simulink model "LQR_s_inv_int"  (R2023b)
settings: Solver=VariableStepAuto  StartTime=0.0  StopTime=10  RelTol=1e-14  AbsTol=1e-20
values from neighbouring files (symbols this model uses):
  K = [k1 k2 ki]    [WP2.m]
undefined symbols (not defined in the file or in its folder): Disturbo
settings Model: Creator=giova  LastModifiedBy=Principale

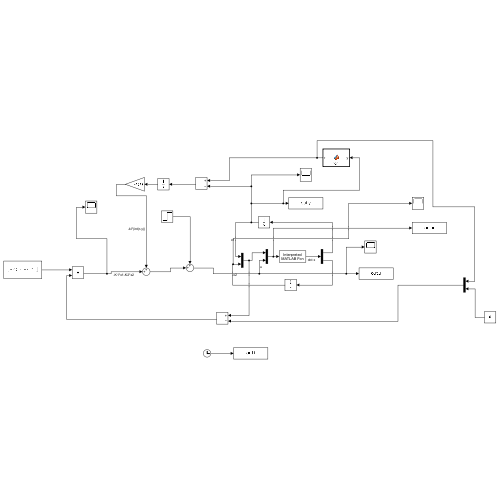
[thumbnail: Simulink's stored preview of the top-level diagram]
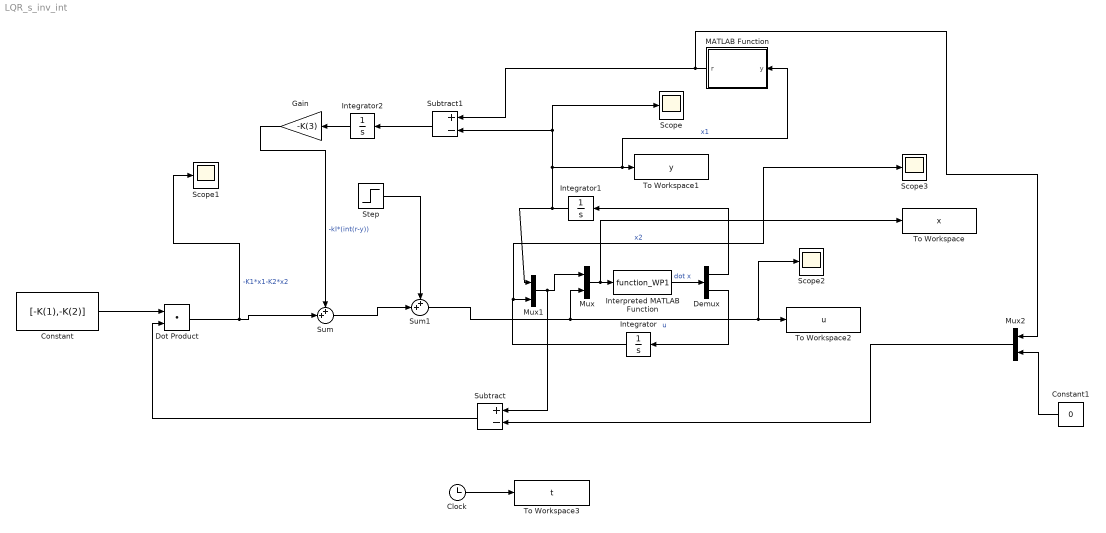
== system LQR_s_inv_int ==
  Clock : Clock
  Constant : Constant  Value=[-K(1),-K(2)]
  Constant1 : Constant  Value=0
  Demux : Demux  Outputs=2
  Dot Product : DotProduct  OutDataTypeStr=Inherit: Inherit via internal rule
  Gain : Gain  Gain=-K(3)
  Integrator : Integrator
  Integrator1 : Integrator
  Integrator2 : Integrator
  Interpreted MATLAB Function : MATLABFcn  MATLABFcn=function_WP1  OutputDimensions=2
  MATLAB Function : MATLAB Function  TreatAsAtomicUnit=on
  Mux : Mux  Inputs=2
  Mux1 : Mux  Inputs=2
  Mux2 : Mux  Inputs=2
  Scope{,1..3} (4 alike) : Scope
  Step : Step  Time=5  After=Disturbo  SampleTime=0
  Subtract : Sum  Inputs=+-
  Subtract1 : Sum  Inputs=+-
  Sum : Sum  Inputs=++|
  Sum1 : Sum  Inputs=++|
  To Workspace : ToWorkspace  VariableName=x  SampleTime=-1
  To Workspace1 : ToWorkspace  VariableName=y  SampleTime=-1
  To Workspace2 : ToWorkspace  VariableName=u  SampleTime=-1
  To Workspace3 : ToWorkspace  VariableName=t  SampleTime=-1
  wires:
  Dot Product/1 -> Sum/2, Scope1/1  "-K1*x1-K2*x2"
  Constant/1 -> Dot Product/1
  Integrator/1 -> Scope3/1, Mux1/2  "x2"
  Demux/2 -> Integrator/1
  Mux1/1 -> Subtract/1, Mux/1
  Clock/1 -> To Workspace3/1
  Subtract/1 -> Dot Product/2
  Integrator1/1 -> Scope/1, Subtract1/2, MATLAB Function/1(y), To Workspace1/1, Mux1/1  "x1"
  Demux/1 -> Integrator1/1
  Mux/1 -> To Workspace/1, Interpreted MATLAB Function/1
  Interpreted MATLAB Function/1 -> Demux/1  "dot x"
  Sum/1 -> Sum1/2
  Sum1/1 -> Mux/2, Scope2/1, To Workspace2/1  "u"
  Subtract1/1 -> Integrator2/1
  Integrator2/1 -> Gain/1
  Gain/1 -> Sum/1  "-kI*(int(r-y))"
  Constant1/1 -> Mux2/2
  Mux2/1 -> Subtract/2
  Step/1 -> Sum1/1
  MATLAB Function/1(r) -> Mux2/1, Subtract1/1

== matlab function LQR_s_inv_int/MATLAB Function ==
  data: y input; r output
function r = fcn(y)
    if(y==0)
        r=pi;
    else
        r=fix(y/(2*pi))*2*pi + pi*sign(y);
    end
end
